simulink model "Modelisation_0_Erreur_de_derivee_numerique"  (R2016a)
settings: Solver=FixedStepAuto  StartTime=0.0  StopTime=10  FixedStep=0.01  MaxStep=0.001  RelTol=1e-3
settings Model: Creator=user  LastModifiedBy=nadour
settings DataIOCC: LimitDataPoints=on  SaveFormat=Array
settings HardwareCC: ProdBitPerPointer=32  ProdLargestAtomicFloat=None  ProdIntDivRoundTo=Undefined  ProdEndianess=Unspecified  ProdWordSize=32  ProdHWDeviceType=32-bit Generic
settings ModelReferenceCC: PropagateSignalLabelsOutOfModel=off
settings ConfigComp: CovModelRefEnable=Off

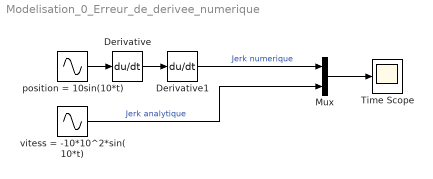
== system Modelisation_0_Erreur_de_derivee_numerique ==
  Derivative : Derivative
  Derivative1 : Derivative
  Mux : Mux  Inputs=2
  Time Scope : Scope
  position = 10sin(10*t) : Sin  Amplitude=10  Frequency=10  SampleTime=0
  vitess = -10*10^2*sin(10*t) : Sin  Amplitude=-10*10^2  Frequency=10  SampleTime=0
  wires:
  Derivative/1 -> Derivative1/1
  Derivative1/1 -> Mux/1  "Jerk numerique"
  position = 10sin(10*t)/1 -> Derivative/1
  vitess = -10*10^2*sin(10*t)/1 -> Mux/2  "Jerk analytique"
  Mux/1 -> Time Scope/1
